simulink model "GuytonModel1972WithSubsystems_R2018_new"  (Simulink 9.1)
settings: Solver=ode23tb  StartTime=0.0  StopTime=inf  RelTol=1e-3  EnableMultiTasking=on
(part 2 of 3)

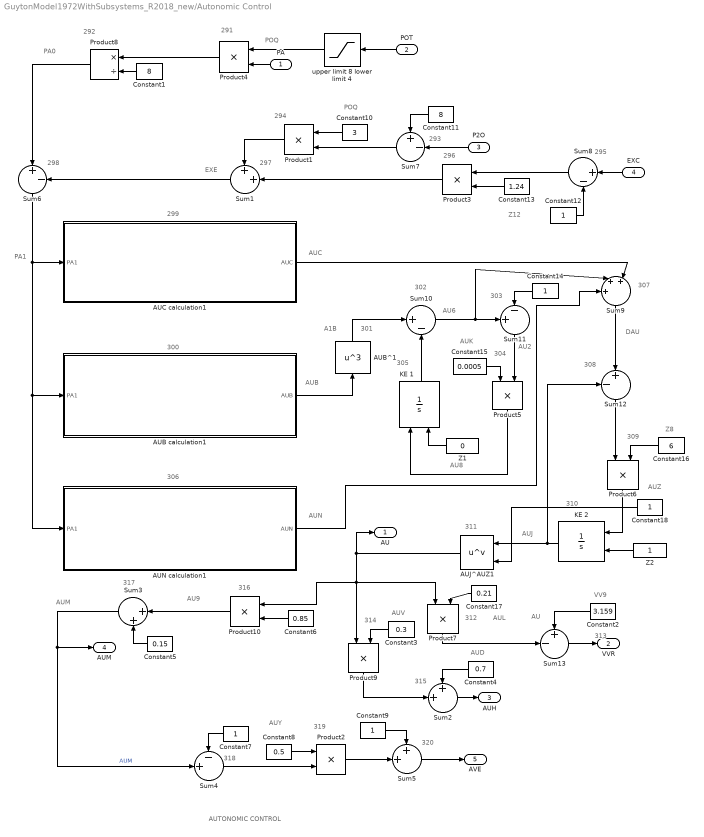
== system GuytonModel1972WithSubsystems_R2018_new/Autonomic Control ==
  note: AU
  note: AUZ
  note: PA0
  note: 306
  note: 300
  note: 294
  note: 293
  note: 305
  note: 299
  note: 297
  note: 315
  note: 295
  note: 302
  note: 309
  note: 298
  note: 314
  note: 311
  note: 301
  note: AUTONOMIC CONTROL
  note: 304
  note: 318
  note: 307
  note: 320
  note: 292
  note: AU6
  note: 316
  note: POQ
  note: DAU
  note: AU8
  note: AUK
  note: 317
  note: 291
  note: AUJ
  note: 296
  note: AUY
  note: 319
  note: 308
  note: A1B
  note: AU9
  note: 312
  note: AUV
  note: AUB
  note: 313
  note: Z12
  note: AUN
  note: AU2
  note: AUL
  note: VV9
  note: 310
  note: Z8
  note: EXE
  note: POQ
  note: 303
  note: AUC
  note: AUD
  note: PA1
  note: AUM
  PA : Inport
  POT : Inport  Port=2
  P2O : Inport  Port=3
  EXC : Inport  Port=4
  AUB calculation1 : Subsystem
      mask Display: disp('AUB CALCULATION \n\nwhen PA1<40: AUB=1.85718             \nwhen  40>PA1<170: AUB=0.014286*(170-PA1)\nwhen PA1>=170: AUB=0               \n')
  AUB^1 : Fcn  Expr=u^3
  AUC calculation1 : Subsystem
      mask Display: disp('AUC CALCULATION \n\nwhen PA1<40: AUC=1.2             \nwhen  40>PA1<80: AUC=0.03*(80-PA1)\nwhen PA1>=80: AUC=0               \n')
  AUJ^AUZ1 : Math  Operator=pow  SaturateOnIntegerOverflow=on
  AUN calculation1 : Subsystem
      mask Display: disp('AUN CALCULATION \n\nwhen PA1<50: AUN=6            \nwhen  20>PA1<50: AUN=0.2*(50-PA1)\nwhen PA1>=50: AUN=0               \n')
  Constant1 : Constant  Value=8
  Constant10 : Constant  Value=3
  Constant11 : Constant  Value=8
  Constant{7,9,12,14,18} (5 alike) : Constant
  Constant13 : Constant  Value=1.24
  Constant15 : Constant  Value=0.0005
  Constant16 : Constant  Value=6
  Constant17 : Constant  Value=0.21
  Constant2 : Constant  Value=3.159
  Constant3 : Constant  Value=0.3
  Constant4 : Constant  Value=0.7
  Constant5 : Constant  Value=0.15
  Constant6 : Constant  Value=0.85
  Constant8 : Constant  Value=0.5
  KE 1 : Integrator  InitialConditionSource=external  InitialCondition=74.7024
  KE 2 : Integrator  InitialConditionSource=external  InitialCondition=74.7024
  Product{1..7,9..10} (9 alike) : Product  SaturateOnIntegerOverflow=on  RndMeth=Zero  InputSameDT=on  OutDataTypeStr=Inherit: Same as first input
  Product8 : Product  Inputs=*/  SaturateOnIntegerOverflow=on  RndMeth=Zero  InputSameDT=on  OutDataTypeStr=Inherit: Same as first input
  Sum1 : Sum  Inputs=++|  SaturateOnIntegerOverflow=on  InputSameDT=on  OutDataTypeStr=Inherit: Same as first input
  Sum10 : Sum  Inputs=|+-  SaturateOnIntegerOverflow=on  InputSameDT=on  OutDataTypeStr=Inherit: Same as first input
  Sum11 : Sum  Inputs=+-|  SaturateOnIntegerOverflow=on  InputSameDT=on  OutDataTypeStr=Inherit: Same as first input
  Sum12 : Sum  Inputs=-+|  SaturateOnIntegerOverflow=on  InputSameDT=on  OutDataTypeStr=Inherit: Same as first input
  Sum13 : Sum  Inputs=+-|  SaturateOnIntegerOverflow=on  InputSameDT=on  OutDataTypeStr=Inherit: Same as first input
  Sum2 : Sum  Inputs=++|  SaturateOnIntegerOverflow=on  InputSameDT=on  OutDataTypeStr=Inherit: Same as first input
  Sum3 : Sum  Inputs=|++  SaturateOnIntegerOverflow=on  InputSameDT=on  OutDataTypeStr=Inherit: Same as first input
  Sum4 : Sum  Inputs=-+|  SaturateOnIntegerOverflow=on  InputSameDT=on  OutDataTypeStr=Inherit: Same as first input
  Sum5 : Sum  Inputs=++|  SaturateOnIntegerOverflow=on  InputSameDT=on  OutDataTypeStr=Inherit: Same as first input
  Sum6 : Sum  Inputs=|+-  SaturateOnIntegerOverflow=on  InputSameDT=on  OutDataTypeStr=Inherit: Same as first input
  Sum7 : Sum  Inputs=+-|  SaturateOnIntegerOverflow=on  InputSameDT=on  OutDataTypeStr=Inherit: Same as first input
  Sum8 : Sum  Inputs=|+-  SaturateOnIntegerOverflow=on  InputSameDT=on  OutDataTypeStr=Inherit: Same as first input
  Sum9 : Sum  Inputs=+++|  SaturateOnIntegerOverflow=on  InputSameDT=on  OutDataTypeStr=Inherit: Same as first input
  Z1 : Constant  Value=0
  Z2 : Constant
  "upper limit 8 lower limit 4 " : Saturate  UpperLimit=8  LowerLimit=4  LinearizeAsGain=off  ZeroCross=off
  AU : Outport
  VVR : Outport  Port=2
  AUH : Outport  Port=3
  AUM : Outport  Port=4
  AVE : Outport  Port=5
  wires:
  Sum7/1 -> Product1/2
  Sum5/1 -> AVE/1
  Sum1/1 -> Sum6/2
  Constant2/1 -> Sum13/1
  Product5/1 -> KE 1/1
  AUB^1/1 -> Sum10/1
  Constant7/1 -> Sum4/1
  Product8/1 -> Sum6/1
  Sum3/1 -> AUM/1, Sum4/2  "AUM"
  Z1/1 -> KE 1/2
  POT/1 -> "upper limit 8 lower limit 4 "/1
  Product4/1 -> Product8/1
  Constant4/1 -> Sum2/1
  Constant18/1 -> AUJ^AUZ1/2
  ? -> ?
  AUB calculation1/1(AUB) -> AUB^1/1
  Sum4/1 -> Product2/2
  Sum11/1 -> Product5/2
  Constant8/1 -> Product2/1
  Sum9/1 -> Sum12/2
  P2O/1 -> Sum7/2
  Constant1/1 -> Product8/2
  Constant9/1 -> Sum5/1
  Constant5/1 -> Sum3/2
  Product9/1 -> Sum2/2
  Constant17/1 -> Product7/2
  Product2/1 -> Sum5/2
  Z2/1 -> KE 2/2
  Constant16/1 -> Product6/2
  KE 2/1 -> Sum12/1, AUJ^AUZ1/1
  Product6/1 -> KE 2/1
  Constant3/1 -> Product9/2
  Sum12/1 -> Product6/1
  Sum6/1 -> AUC calculation1/1(PA1), AUB calculation1/1(PA1), AUN calculation1/1(PA1)
  KE 1/1 -> Sum10/2
  Product7/1 -> Sum13/2
  Constant13/1 -> Product3/2
  Constant6/1 -> Product10/2
  AUN calculation1/1(AUN) -> Sum9/1
  AUC calculation1/1(AUC) -> Sum9/3
  Constant14/1 -> Sum11/2
  Constant15/1 -> Product5/1
  Sum10/1 -> Sum11/1, Sum9/2
  Product1/1 -> Sum1/1
  Product3/1 -> Sum1/2
  AUJ^AUZ1/1 -> AU/1, Product7/1, Product9/1, Product10/1
  Sum8/1 -> Product3/1
  Product10/1 -> Sum3/1
  Constant10/1 -> Product1/1
  Constant12/1 -> Sum8/2
  "upper limit 8 lower limit 4 "/1 -> Product4/1
  Constant11/1 -> Sum7/1
  EXC/1 -> Sum8/1
  PA/1 -> Product4/2
  Sum13/1 -> VVR/1
  Sum2/1 -> AUH/1

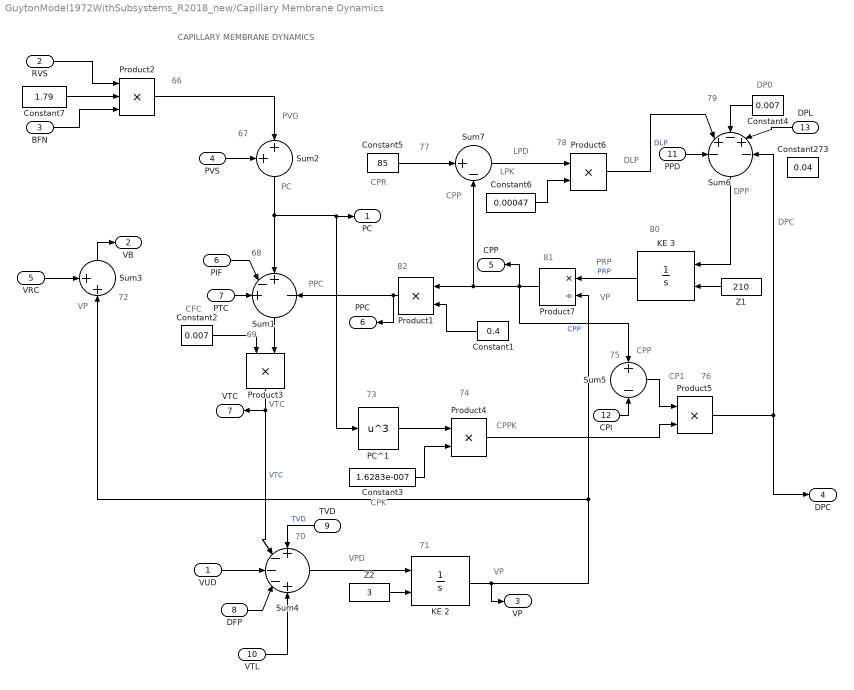
== system GuytonModel1972WithSubsystems_R2018_new/Capillary Membrane Dynamics ==
  note: VTC
  note: 72
  note: 76
  note: 73
  note: 74
  note: 71
  note: 82
  note: 66
  note: 75
  note: 70
  note: 79
  note: CAPILLARY MEMBRANE DYNAMICS
  note: 80
  note: 78
  note: 67
  note: CPPK
  note: PRP
  note: DLP
  note: 81
  note: 77
  note: VP
  note: 69
  note: VPD
  note: DP0
  note: PVG
  note: DPC
  note: CPP
  note: VP
  note: 68
  note: LPK
  note: CPR
  note: PC
  note: CP1
  note: VP
  note: PPC
  note: CPK
  note: DPP
  note: LPD
  note: CFC
  note: CPP
  VUD : Inport
  RVS : Inport  Port=2
  BFN : Inport  Port=3
  PVS : Inport  Port=4
  VRC : Inport  Port=5
  PIF : Inport  Port=6
  PTC : Inport  Port=7
  DFP : Inport  Port=8
  TVD : Inport  Port=9
  VTL : Inport  Port=10
  PPD : Inport  Port=11
  CPI : Inport  Port=12
  DPL : Inport  Port=13
  Constant1 : Constant  Value=0.4
  Constant2 : Constant  Value=0.007
  Constant273 : Constant  Value=0.04
  Constant3 : Constant  Value=1.6283e-007
  Constant4 : Constant  Value=0.007
  Constant5 : Constant  Value=85
  Constant6 : Constant  Value=0.00047
  Constant7 : Constant  Value=1.79
  KE 2 : Integrator  InitialConditionSource=external  InitialCondition=74.7024
  KE 3 : Integrator  InitialConditionSource=external  InitialCondition=74.7024
  PC^1 : Fcn  Expr=u^3
  Product{1,3..6} (5 alike) : Product  SaturateOnIntegerOverflow=on  RndMeth=Zero  InputSameDT=on  OutDataTypeStr=Inherit: Same as first input
  Product2 : Product  Inputs=3  SaturateOnIntegerOverflow=on  RndMeth=Zero  InputSameDT=on  OutDataTypeStr=Inherit: Same as first input
  Product7 : Product  Inputs=*/  SaturateOnIntegerOverflow=on  RndMeth=Zero  InputSameDT=on  OutDataTypeStr=Inherit: Same as first input
  Sum1 : Sum  Inputs=+-+|-  SaturateOnIntegerOverflow=on  InputSameDT=on  OutDataTypeStr=Inherit: Same as first input
  Sum2 : Sum  Inputs=++|  SaturateOnIntegerOverflow=on  InputSameDT=on  OutDataTypeStr=Inherit: Same as first input
  Sum3 : Sum  Inputs=++|  SaturateOnIntegerOverflow=on  InputSameDT=on  OutDataTypeStr=Inherit: Same as first input
  Sum4 : Sum  Inputs=+---+  SaturateOnIntegerOverflow=on  InputSameDT=on  OutDataTypeStr=Inherit: Same as first input
  Sum5 : Sum  Inputs=+|-  SaturateOnIntegerOverflow=on  InputSameDT=on  OutDataTypeStr=Inherit: Same as first input
  Sum6 : Sum  Inputs=-+-+-  SaturateOnIntegerOverflow=on  InputSameDT=on  OutDataTypeStr=Inherit: Same as first input
  Sum7 : Sum  Inputs=|+-  SaturateOnIntegerOverflow=on  InputSameDT=on  OutDataTypeStr=Inherit: Same as first input
  Z1 : Constant  Value=210
  Z2 : Constant  Value=3
  PC : Outport
  VB : Outport  Port=2
  VP : Outport  Port=3
  DPC : Outport  Port=4
  CPP : Outport  Port=5
  PPC : Outport  Port=6
  VTC : Outport  Port=7
  wires:
  Sum3/1 -> VB/1
  Product5/1 -> DPC/1, Sum6/5
  Product2/1 -> Sum2/2
  Product4/1 -> Product5/2
  DPL/1 -> Sum6/4
  Product7/1 -> Product1/1, Sum7/2, Sum5/1, CPP/1  "CPP"
  Sum5/1 -> Product5/1
  VRC/1 -> Sum3/1
  Z1/1 -> KE 3/2
  Constant5/1 -> Sum7/1
  Sum7/1 -> Product6/1
  Constant6/1 -> Product6/2
  Sum6/1 -> KE 3/1
  VTL/1 -> Sum4/5
  PC^1/1 -> Product4/1
  Sum4/1 -> KE 2/1
  Product6/1 -> Sum6/2  "DLP"
  Sum1/1 -> Product3/2
  Product1/1 -> PPC/1, Sum1/4
  Constant2/1 -> Product3/1
  Z2/1 -> KE 2/2
  CPI/1 -> Sum5/2
  Constant3/1 -> Product4/2
  Constant7/1 -> Product2/2
  Product3/1 -> Sum4/2, VTC/1  "VTC"
  Sum2/1 -> Sum1/3, PC/1, PC^1/1
  TVD/1 -> Sum4/1  "TVD"
  BFN/1 -> Product2/3
  KE 2/1 -> VP/1, Product7/2, Sum3/2
  PVS/1 -> Sum2/1
  KE 3/1 -> Product7/1  "PRP"
  Constant1/1 -> Product1/2
  Constant4/1 -> Sum6/3
  RVS/1 -> Product2/1
  PIF/1 -> Sum1/2
  PTC/1 -> Sum1/1
  VUD/1 -> Sum4/3
  DFP/1 -> Sum4/4
  PPD/1 -> Sum6/1

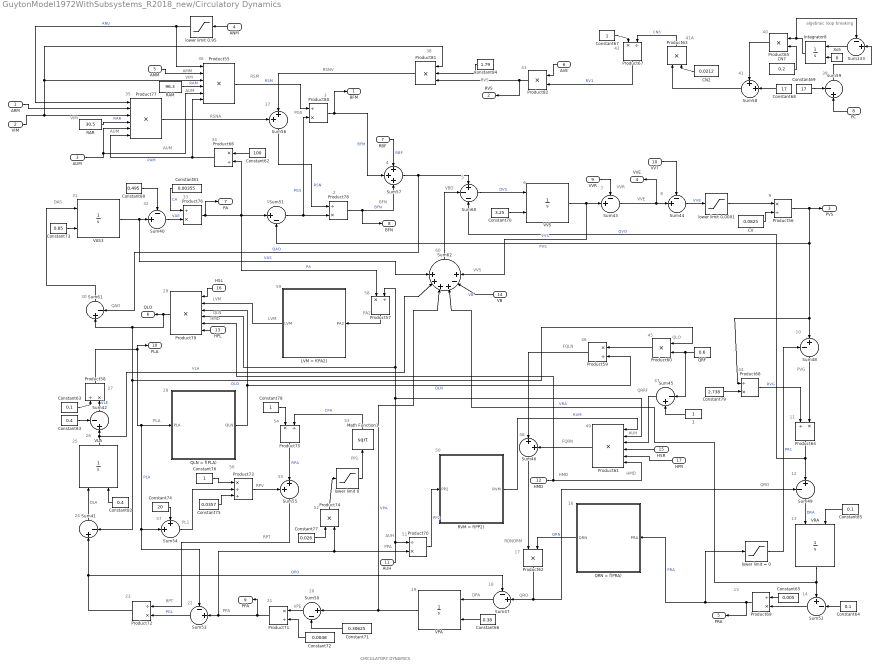
== system GuytonModel1972WithSubsystems_R2018_new/Circulatory Dynamics ==
  note: 24
  note: 25
  note: 30
  note: 58
  note: QLO
  note: AUM
  note: AUM
  note: VIM
  note: BFN
  note: 4
  note: PGS
  note: 38
  note: 39
  note: 6
  note: QLN
  note: 37
  note: AUM
  note: VBD
  note: 50
  note: VVE
  note: 16
  note: QAO
  note: 26
  note: PLA
  note: 41A
  note: 41
  note: 8
  note: 29
  note: 27
  note: 35
  note: 42
  note: 1
  note: PA2
  note: RVS
  note: 5
  note: VIM
  note: RSM
  note: 60
  note: DAS
  note: 33
  note: 31
  note: 9
  note: 59
  note: VVS
  note: 43
  note: 34
  note: 28
  note: 2
  note: 3
  note: 36
  note: 40
  note: LVM
  note: HMD
  note: RPV
  note: 46
  note: 44
  note: 7
  note: PP1
  note: 55
  note: 56
  note: 32
  note: 23
  note: 21
  note: 20
  note: 11
  note: 15
  note: 18
  note: 48
  note: QRO
  note: 22
  note: QRO
  note: VPE
  note: 54
  note: RPT
  note: 51
  note: RPT
  note: 12
  note: PL1
  note: LVM
  note: 14
  note: 45
  note: AMM
  note: 47
  note: HMD
  note: 49
  note: HMD
  note: 13
  note: VVR
  note: PPA
  note: 57
  note: AUH
  note: CIRCULATORY DYNAMICS
  note: 52
  note: 19
  note: PVG
  note: DPA
  note: RSNV
  note: AUH
  note: FQLN
  note: PPA
  note: algebraic
      | loop
      | breaking
  note: 10
  note: QRRF
  note: RDNORM
  note: 17
  note: 53
  note: FQRN
  note: RSNA
  ARM : Inport
  VIM : Inport  Port=2
  AUM : Inport  Port=3
  ANM : Inport  Port=4
  AMM : Inport  Port=5
  AVE : Inport  Port=6
  RBF : Inport  Port=7
  PC : Inport  Port=8
  VVR : Inport  Port=9
  VV7 : Inport  Port=10
  AUH : Inport  Port=11
  HMD : Inport  Port=12
  HPL : Inport  Port=13
  VB : Inport  Port=14
  HSR : Inport  Port=15
  HSL : Inport  Port=16
  HPR : Inport  Port=17
  " VAS3" : Integrator  InitialConditionSource=external
  " VLA" : Integrator  InitialConditionSource=external
  " VPA" : Integrator  InitialConditionSource=external
  " VRA" : Integrator  InitialConditionSource=external
  " VVS" : Integrator  InitialConditionSource=external
  "1 " : Constant
  CN2 : Constant  Value=0.0212
  CN7 : Constant  Value=0.2
  CV : Constant  Value=0.0825
  Constant62 : Constant  Value=100
  Constant63 : Constant  Value=0.1
  Constant64 : Constant  Value=0.1
  Constant65 : Constant  Value=0.005
  Constant66 : Constant  Value=0.38
  Constant67 : Constant
  Constant68 : Constant  Value=17
  Constant69 : Constant  Value=17
  Constant70 : Constant  Value=3.25
  Constant71 : Constant  Value=0.30625
  Constant72 : Constant  Value=0.0048
  Constant73 : Constant  Value=0.85
  Constant74 : Constant  Value=20
  Constant75 : Constant  Value=0.0357
  Constant76 : Constant
  Constant77 : Constant  Value=0.026
  Constant78 : Constant
  Constant79 : Constant  Value=2.738
  Constant80 : Constant  Value=0.495
  Constant81 : Constant  Value=0.00355
  Constant82 : Constant  Value=0.4
  Constant83 : Constant  Value=0.4
  Constant84 : Constant  Value=1.79
  Constant85 : Constant  Value=0.1
  Integrator8 : Integrator  InitialConditionSource=external
  LVM = f(PA2) : Subsystem
      mask Display:
      | plot([0 2.1 4.2 6.3 8.4 10.5 12.6 14.7 16.8 18.9 21 23.1 25.2 27.3 29.4 31.5 33.6 35.7 37.8 39.9 42 44.1 46.2 48.3 50.4 52.5 54.6 56.7 58.8 60.9 63 65.1 67.2 69.3 71.4 73.5 75.6 77.7 79.8 81.9 84 86.1 88.2 90.3 92.4 94.5 96.6 98.7 100.8 102.9 105 107.1 109.2 111.3 113.4 115.5 117.6 119.7 121.8 123.9 126 128.1 130.2 132.3 134.4 136.5 138.6 140.7 142.8 144.9 147 149.1 151.2 153.3 155.4 157.5 159.6 161.7 163.8 165.9 168 170.1 172.2 174.3 176.4 178.5 180.6 182.7 184.8 186.9 189 191.1 193.2 195.3 197.4 199.5 201.6 203.7 205.8 207.9 210 212.1 214.2 216.3 218.4 220.5 222.6 224.7 226.8 228.9 231 233.1 235.2 237.3 239.4], [1.04 1.03998 1.03993 1.03985 1.03973 1.03958 1.03941 1.0392 1.03896 1.03869 1.03839 1.03807 1.03772 1.03734 1.03693 1.03651 1.03605 1.03558 1.03508 1.03455 1.03401 1.03345 1.03286 1.03225 1.03163 1.03099 1.03033 1.02965 1.02895 1.02824 1.02752 1.02678 1.02603 1.02526 1.02443 1.0234 1.02218 1.02078 1.01923 1.01753 1.01572 1.01381 1.01181 1.00976 1.00766 1.00554 1.00341 1.00129 0.999208 0.997118 0.994998 0.992831 0.9906 0.988287 0.985875 0.983347 0.980687 0.977876 0.974898 0.971736 0.968374 0.964817 0.961055 0.95708 0.952882 0.948451 0.943777 0.93885 0.93366 0.928197 0.922452 0.916415 0.910075 0.903423 0.89645 0.889144 0.881496 0.873291 0.86413 0.854038 0.84305 0.831201 0.818528 0.805065 0.790848 0.775913 0.760295 0.744029 0.727152 0.709697 0.691702 0.673201 0.65423 0.634825 0.61502 0.594852 0.574045 0.551912 0.528467 0.503753 0.477816 0.4507 0.422449 0.393107 0.362719 0.33133 0.298983 0.265724 0.231596 0.196644 0.160913 0.124446 0.087288 0.0494838 0.0110776])
      | 
      | text(-30,0.5,'')
      | text(260,0.5,'')
      | text(25,1.15,'')
      | text(25,-0.1,'')
      | text(-25,0.05,'0')
      | text(10,-0.04,'0')
      | text(-25,1.1,'1.4')
      | text(218,-0.04,'260')
  Math Function1 : Math  Operator=sqrt  SaturateOnIntegerOverflow=on
  Product{55,61,77,79} (4 alike) : Product  Inputs=6  SaturateOnIntegerOverflow=on  RndMeth=Zero  InputSameDT=on  OutDataTypeStr=Inherit: Same as first input
  Product{56..57,59,66..67,71,75} (7 alike) : Product  Inputs=*/  SaturateOnIntegerOverflow=on  RndMeth=Zero  InputSameDT=on  OutDataTypeStr=Inherit: Same as first input
  Product{58,64,68..70,72,76,78,80} (9 alike) : Product  Inputs=/*  SaturateOnIntegerOverflow=on  RndMeth=Zero  InputSameDT=on  OutDataTypeStr=Inherit: Same as first input
  Product{60,62..63,65,74,82} (6 alike) : Product  SaturateOnIntegerOverflow=on  RndMeth=Zero  InputSameDT=on  OutDataTypeStr=Inherit: Same as first input
  Product73 : Product  Inputs=*//  SaturateOnIntegerOverflow=on  RndMeth=Zero  InputSameDT=on  OutDataTypeStr=Inherit: Same as first input
  Product81 : Product  Inputs=3  SaturateOnIntegerOverflow=on  RndMeth=Zero  InputSameDT=on  OutDataTypeStr=Inherit: Same as first input
  QLN = f(PLA) : Subsystem
      mask Display:
      | plot([     -5 -4 -3 -2 -1 0 1 2 3 4 5 6 7 8 9 10 11 12 13 14 15 16 17 18 19 20], [ 0 0.01 0.65885 2.08416 3.6 5.05 6.60577 8.16154 9.4 10.2738 10.9872 11.6 12.2245 12.8412 13.3123 13.5 13.5 13.5 13.5 13.5 13.5 13.5 13.5 13.5 13.5 13.5] )
      | 
      | 
      | text(-8,10,'')
      | text(10,-1.5,'')
      | text(22,10,'')
      | text(16,16,'')
      | text(-7,1,'0')
      | text(-5,-0.8,'-4')
      | text(-7,15,'15')
      | text(18,0,'20')
  QRF : Constant  Value=0.6
  QRN = f(PRA) : Subsystem
      mask Display:
      | plot([     -6 -5 -4 -3 -2 -1 0 1 2 3 4 5 6 7 8 9 10 11 12 13 14 15 16 17 18 19 20], [0 0.103491 0.373648 0.75 1.42618 2.6 5 7.61127 9.8 11.1961 12.1 12.6396 13.0852 13.3882 13.5 13.5 13.5 13.5 13.5 13.5 13.5 13.5 13.5 13.5 13.5 13.5 13.5])
      | 
      | 
      | 
      | text(-8,10,'')
      | text(10,-1.5,'')
      | text(22,10,'')
      | text(16,16,'')
      | text(-7,1,'0')
      | text(-5,-0.8,'-4')
      | text(-7,15,'15')
      | text(18,0,'20')
  RAM : Constant  Value=96.3
  RAR : Constant  Value=30.5
  RVM = f(PP2) : Subsystem
      mask Display:
      | plot([0 2.5 5 7.5 10 12.5 15 17.5 20 22.5 25 27.5 30 32.5 35 37.5 40 42.5 45], [1.06 1.05508 1.04813 1.03961 1.03 1.01865 1.00472 0.988437 0.97 0.947748 0.915021 0.864829 0.8 0.715601 0.608483 0.485782 0.347126 0.183428 5.55112e-017])
      | 
      | text(-8,0.5,'')
      | text(50,0.5,'')
      | text(25,1.15,'')
      | text(25,-0.1,'')
      | text(-7,0.05,'0')
      | text(-2,-0.04,'0')
      | text(-7,1.1,'1.4')
      | text(44,-0.04,'50')
  Sum{40,42..44,47..49,53,59,133} (10 alike) : Sum  Inputs=-+|  SaturateOnIntegerOverflow=on  InputSameDT=on  OutDataTypeStr=Inherit: Same as first input
  Sum{41,50..51,61} (4 alike) : Sum  Inputs=|+-  SaturateOnIntegerOverflow=on  InputSameDT=on  OutDataTypeStr=Inherit: Same as first input
  Sum45 : Sum  Inputs=|-+  SaturateOnIntegerOverflow=on  InputSameDT=on  OutDataTypeStr=Inherit: Same as first input
  Sum46 : Sum  Inputs=|++  SaturateOnIntegerOverflow=on  InputSameDT=on  OutDataTypeStr=Inherit: Same as first input
  Sum52 : Sum  Inputs=+-|  SaturateOnIntegerOverflow=on  InputSameDT=on  OutDataTypeStr=Inherit: Same as first input
  Sum{54..56,58} (4 alike) : Sum  Inputs=++|  SaturateOnIntegerOverflow=on  InputSameDT=on  OutDataTypeStr=Inherit: Same as first input
  Sum57 : Sum  Inputs=+++  SaturateOnIntegerOverflow=on  InputSameDT=on  OutDataTypeStr=Inherit: Same as first input
  Sum60 : Sum  Inputs=+--  SaturateOnIntegerOverflow=on  InputSameDT=on  OutDataTypeStr=Inherit: Same as first input
  Sum62 : Sum  Inputs=++++-+  SaturateOnIntegerOverflow=on  InputSameDT=on  OutDataTypeStr=Inherit: Same as first input
  Xo5 : Constant  Value=0  VectorParams1D=off
  "lower limit 0 " : Saturate  UpperLimit=inf  LowerLimit=0  LinearizeAsGain=off
  lower limit 0.0001 : Saturate  UpperLimit=inf  LowerLimit=0.0001  LinearizeAsGain=off
  lower limit 0.95 : Saturate  UpperLimit=inf  LowerLimit=0.95  LinearizeAsGain=off
  lower limit = 0 : Saturate  UpperLimit=inf  LowerLimit=0  LinearizeAsGain=off
  BFM : Outport
  RVS : Outport  Port=2
  PVS : Outport  Port=3
  VVE : Outport  Port=4
  PRA : Outport  Port=5
  QLO : Outport  Port=6
  PA : Outport  Port=7
  BFN : Outport  Port=8
  PPA : Outport  Port=9
  PLA : Outport  Port=10
  wires:
  "1 "/1 -> Sum45/2
  lower limit 0.95/1 -> Product77/1, Product55/1  "ANU"
  QRF/1 -> Product60/2, Sum45/1
  Product58/1 -> PLA/1, Sum54/2, Sum53/1, QLN = f(PLA)/1(PLA)  "PLA"
  Product76/1 -> PA/1, Sum51/1, Product57/1, Product66/2  "PA"
  Product59/1 -> Sum46/1
  Integrator8/1 -> Product65/1, Sum133/1
  Constant77/1 -> Product74/1
  Xo5/1 -> Integrator8/2
  Sum59/1 -> Sum133/2
  Sum46/1 -> Product62/1
  HMD/1 -> Product61/6, Product79/5
  AUH/1 -> Product57/2, Product79/4, Product61/2, Product70/1
  Sum54/1 -> Product73/2
  Sum133/1 -> Integrator8/1
  lower limit = 0/1 -> Sum48/1  "PR1"
  Product69/1 -> PRA/1, lower limit = 0/1, QRN = f(PRA)/1(PRA)  "PRA"
  Constant63/1 -> Product58/1
  Product70/1 -> RVM = f(PP2)/1(PP2)  "PP2"
  Constant71/1 -> Sum50/2
  Product71/1 -> PPA/1, Product70/2, Product74/2, Sum53/2
  " VRA"/1 -> Sum52/1, Sum62/4  "VRA"
  Constant79/1 -> Product68/2
  Constant78/1 -> Product75/1
  Sum45/1 -> Product61/3
  " VLA"/1 -> Sum42/2, Sum62/2  "VLA"
  Sum41/1 -> " VLA"/1  "DLA"
  Constant82/1 -> " VLA"/2
  "lower limit 0 "/1 -> Math Function1/1
  Sum60/1 -> " VVS"/1  "DVS"
  QLN = f(PLA)/1(QLN) -> Product59/2, Product79/3  "QLN"
  Sum58/1 -> Product63/1
  Constant68/1 -> Sum58/2
  CV/1 -> Product56/2
  Sum43/1 -> Sum44/2, VVE/1
  CN7/1 -> Product65/2
  Product65/1 -> Sum58/1
  RVM = f(PP2)/1(RVM) -> Product61/1  "RVM"
  Sum44/1 -> lower limit 0.0001/1  "VV8"
  Product80/1 -> BFM/1, Sum57/2  "BFM"
  Product67/1 -> Product82/2  "RV1"
  Product79/1 -> Sum61/1, Product60/1, Sum41/2, QLO/1  "QLO"
  ANM/1 -> lower limit 0.95/1
  Product63/1 -> Product67/2  "CN3"
  Sum40/1 -> Product76/2  "VAE"
  Product66/1 -> Product77/6, Product55/6  "PAM"
  Product81/1 -> Sum56/2
  Sum48/1 -> Product64/2
  Constant64/1 -> Sum52/2
  Constant70/1 -> " VVS"/2
  Sum52/1 -> Product69/2
  Product74/1 -> "lower limit 0 "/1
  Constant66/1 -> " VPA"/2
  Sum55/1 -> Product72/1
  Sum57/1 -> Sum60/1, Sum61/2  "QAO"
  Constant80/1 -> Sum40/1
  RAM/1 -> Product55/4  "RAM"
  Product61/1 -> Sum46/2
  Sum53/1 -> Product72/2  "PGL"
  Constant84/1 -> Product81/2
  Product68/1 -> Product64/1  "RVG"
  Product57/1 -> LVM = f(PA2)/1(PA2)
  Product78/1 -> BFN/1, Sum57/3  "BFN"
  CN2/1 -> Product63/2
  Constant67/1 -> Product67/1
  Constant81/1 -> Product76/1  "CA"
  AMM/1 -> Product55/2
  Constant65/1 -> Product69/1
  VVR/1 -> Sum43/1
  Sum51/1 -> Product78/2, Product80/2  "PGS"
  QRN = f(PRA)/1(QRN) -> Product62/2  "QRN"
  AUM/1 -> Product77/5, Product55/5
  ARM/1 -> Product77/2
  Sum62/1 -> Sum60/2
  Constant72/1 -> Product71/2
  RAR/1 -> Product77/4  "RAR"
  Constant83/1 -> Sum42/1
  Constant75/1 -> Product73/3
  Product72/1 -> Sum41/1, Sum47/1  "QPO"
  Math Function1/1 -> Product75/2  "CPA"
  Product60/1 -> Product59/1
  lower limit 0.0001/1 -> Product56/1
  Constant62/1 -> Product66/1
  Product82/1 -> RVS/1, Product81/3
  LVM = f(PA2)/1(LVM) -> Product79/2
  Sum49/1 -> " VRA"/1  "DRA"
  Constant76/1 -> Product73/1
  Sum42/1 -> Product58/2  "VLE"
  Sum50/1 -> Product71/1
  " VAS3"/1 -> Sum40/2, Sum62/1  "VAS"
  Product77/1 -> Sum56/1
  Sum47/1 -> " VPA"/1
  " VPA"/1 -> Sum50/1, Sum62/3  "VPA"
  Constant69/1 -> Sum59/1
  Product55/1 -> Product80/1  "RSM"
  Constant85/1 -> " VRA"/2
  VIM/1 -> Product77/3, Product81/1, Product55/3
  VB/1 -> Sum62/5  "VB"
  Product56/1 -> PVS/1, Sum51/2, Sum48/2, Product68/1  "PVS"
  Product64/1 -> Sum60/3, Sum49/2  "QVO"
  " VVS"/1 -> Sum62/6, Sum43/2  "VVS"
  Constant73/1 -> " VAS3"/2
  Product75/1 -> Sum55/2  "RPA"
  Sum61/1 -> " VAS3"/1
  Sum56/1 -> Product78/1  "RSN"
  Product62/1 -> Sum47/2, Sum49/1
  RBF/1 -> Sum57/1  "RBF"
  Product73/1 -> Sum55/1
  Constant74/1 -> Sum54/1
  HSL/1 -> Product79/1
  HSR/1 -> Product61/4
  HPR/1 -> Product61/5
  AVE/1 -> Product82/1
  VV7/1 -> Sum44/1
  HPL/1 -> Product79/6
  PC/1 -> Sum59/2

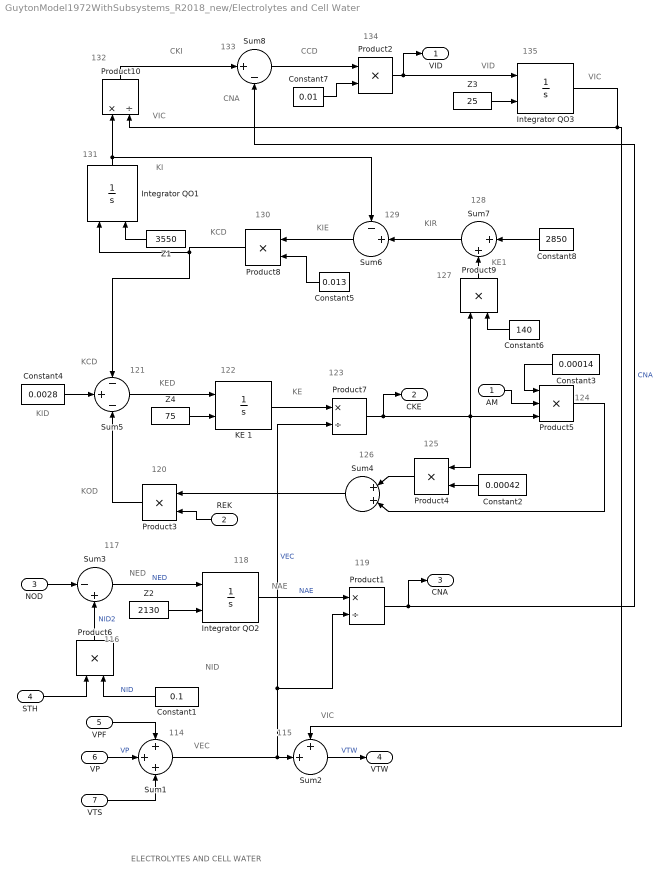
== system GuytonModel1972WithSubsystems_R2018_new/Electrolytes and Cell Water ==
  note: 132
  note: 124
  note: 129
  note: 130
  note: CKI
  note: VID
  note: KI
  note: 114
  note: VIC
  note: 122
  note: 125
  note: KE
  note: 117
  note: KCD
  note: ELECTROLYTES AND CELL WATER
  note: 115
  note: KCD
  note: 134
  note: 119
  note: KID
  note: 118
  note: VIC
  note: 121
  note: KE1
  note: 120
  note: 131
  note: CCD
  note: CNA
  note: KIE
  note: 116
  note: NAE
  note: VIC
  note: 127
  note: VEC
  note: KIR
  note: KOD
  note: NED
  note: NID
  note: 128
  note: 135
  note: 123
  note: KED
  note: 126
  note: 133
  AM : Inport
  REK : Inport  Port=2
  NOD : Inport  Port=3
  STH : Inport  Port=4
  VPF : Inport  Port=5
  VP : Inport  Port=6
  VTS : Inport  Port=7
  Constant1 : Constant  Value=0.1
  Constant2 : Constant  Value=0.00042
  Constant3 : Constant  Value=0.00014
  Constant4 : Constant  Value=0.0028
  Constant5 : Constant  Value=0.013
  Constant6 : Constant  Value=140
  Constant7 : Constant  Value=0.01
  Constant8 : Constant  Value=2850
  Integrator QO1 : Integrator  InitialConditionSource=external  InitialCondition=2403.143066
  Integrator QO2 : Integrator  InitialConditionSource=external  InitialCondition=2403.143066
  Integrator QO3 : Integrator  InitialConditionSource=external  InitialCondition=2403.143066
  KE 1 : Integrator  InitialConditionSource=external  InitialCondition=74.7024
  Product1 : Product  Inputs=*/  SaturateOnIntegerOverflow=on  RndMeth=Zero  InputSameDT=on  OutDataTypeStr=Inherit: Same as first input
  Product10 : Product  Inputs=*/  SaturateOnIntegerOverflow=on  RndMeth=Zero  InputSameDT=on  OutDataTypeStr=Inherit: Same as first input
  Product{2..4,6,8..9} (6 alike) : Product  SaturateOnIntegerOverflow=on  RndMeth=Zero  InputSameDT=on  OutDataTypeStr=Inherit: Same as first input
  Product5 : Product  Inputs=3  SaturateOnIntegerOverflow=on  RndMeth=Zero  InputSameDT=on  OutDataTypeStr=Inherit: Same as first input
  Product7 : Product  Inputs=*/  SaturateOnIntegerOverflow=on  RndMeth=Zero  InputSameDT=on  OutDataTypeStr=Inherit: Same as first input
  Sum1 : Sum  Inputs=+++  SaturateOnIntegerOverflow=on  InputSameDT=on  OutDataTypeStr=Inherit: Same as first input
  Sum2 : Sum  Inputs=++|  SaturateOnIntegerOverflow=on  InputSameDT=on  OutDataTypeStr=Inherit: Same as first input
  Sum3 : Sum  Inputs=|-+  SaturateOnIntegerOverflow=on  InputSameDT=on  OutDataTypeStr=Inherit: Same as first input
  Sum4 : Sum  Inputs=|++|  SaturateOnIntegerOverflow=on  InputSameDT=on  OutDataTypeStr=Inherit: Same as first input
  Sum5 : Sum  Inputs=-+-  SaturateOnIntegerOverflow=on  InputSameDT=on  OutDataTypeStr=Inherit: Same as first input
  Sum6 : Sum  Inputs=-+|  SaturateOnIntegerOverflow=on  InputSameDT=on  OutDataTypeStr=Inherit: Same as first input
  Sum7 : Sum  Inputs=|++  SaturateOnIntegerOverflow=on  InputSameDT=on  OutDataTypeStr=Inherit: Same as first input
  Sum8 : Sum  Inputs=|+-  SaturateOnIntegerOverflow=on  InputSameDT=on  OutDataTypeStr=Inherit: Same as first input
  Z1 : Constant  Value=3550
  Z2 : Constant  Value=2130
  Z3 : Constant  Value=25
  Z4 : Constant  Value=75
  VID : Outport
  CKE : Outport  Port=2
  CNA : Outport  Port=3
  VTW : Outport  Port=4
  wires:
  Product3/1 -> Sum5/3
  Product5/1 -> Sum4/2
  Constant4/1 -> Sum5/2
  Sum4/1 -> Product3/1
  Z3/1 -> Integrator QO3/2
  Constant6/1 -> Product9/2
  Product6/1 -> Sum3/2  "NID2"
  Z4/1 -> KE 1/2
  Constant5/1 -> Product8/2
  Constant7/1 -> Product2/2
  Product2/1 -> VID/1, Integrator QO3/1
  Constant2/1 -> Product4/2
  Constant8/1 -> Sum7/1
  Z2/1 -> Integrator QO2/2
  Sum3/1 -> Integrator QO2/1  "NED"
  Sum6/1 -> Product8/1
  Integrator QO3/1 -> Sum2/1, Product10/2
  Sum7/1 -> Sum6/2
  Integrator QO1/1 -> Sum6/1, Product10/1
  KE 1/1 -> Product7/1
  Sum5/1 -> KE 1/1
  Constant1/1 -> Product6/2  "NID"
  Z1/1 -> Integrator QO1/2
  Product7/1 -> CKE/1, Product4/1, Product5/3, Product9/1
  Constant3/1 -> Product5/1
  Product1/1 -> CNA/1, Sum8/2  "CNA"
  Sum2/1 -> VTW/1  "VTW"
  Product4/1 -> Sum4/1
  Integrator QO2/1 -> Product1/1  "NAE"
  Sum8/1 -> Product2/1
  Product10/1 -> Sum8/1
  NOD/1 -> Sum3/1
  VP/1 -> Sum1/2  "VP"
  Product8/1 -> Integrator QO1/1, Sum5/1
  Product9/1 -> Sum7/2
  Sum1/1 -> Product1/2, Product7/2, Sum2/2  "VEC"
  VTS/1 -> Sum1/3
  VPF/1 -> Sum1/1
  STH/1 -> Product6/1
  REK/1 -> Product3/2
  AM/1 -> Product5/2

== system GuytonModel1972WithSubsystems_R2018_new/Heart Hypertrophy or Deterioration ==
  note: HPR
  note: 340
  note: 347
  note: 345
  note: 342
  note: 343
  note: 348
  note: 350
  note: 351
  note: HPL
  note: DHM
  note: 352
  note: HEART HYPERTROPHY OR DETERIORATION
  note: 346
  note: 344
  note: PPA4
  note: HPL
  note: 349
  note: 341
  note: PP3
  PA : Inport
  PPA : Inport  Port=2
  HSL : Inport  Port=3
  POT : Inport  Port=4
  HSR : Inport  Port=5
  Constant1 : Constant  Value=100
  Constant2 : Constant  Value=57600
  Constant3 : Constant  Value=15
  Constant4 : Constant  Value=57600
  Constant5 : Constant  Value=6
  Constant6 : Constant  Value=0.0025
  KE 1 : Integrator  InitialConditionSource=external  InitialCondition=74.7024
  KE 2 : Integrator  InitialConditionSource=external  InitialCondition=74.7024
  KE 3 : Integrator  InitialConditionSource=external  InitialCondition=74.7024
  PA4^0.1 : Fcn  Expr=u^0.625
  PP3^0.2 : Fcn  Expr=u^0.625
  Product1 : Product  Inputs=*/  SaturateOnIntegerOverflow=on  RndMeth=Zero  InputSameDT=on  OutDataTypeStr=Inherit: Same as first input
  Product2 : Product  Inputs=/*/  SaturateOnIntegerOverflow=on  RndMeth=Zero  InputSameDT=on  OutDataTypeStr=Inherit: Same as first input
  Product3 : Product  Inputs=*/  SaturateOnIntegerOverflow=on  RndMeth=Zero  InputSameDT=on  OutDataTypeStr=Inherit: Same as first input
  Product4 : Product  SaturateOnIntegerOverflow=on  RndMeth=Zero  InputSameDT=on  OutDataTypeStr=Inherit: Same as first input
  Product5 : Product  Inputs=/*/  SaturateOnIntegerOverflow=on  RndMeth=Zero  InputSameDT=on  OutDataTypeStr=Inherit: Same as first input
  Sum1 : Sum  Inputs=|+-  SaturateOnIntegerOverflow=on  InputSameDT=on  OutDataTypeStr=Inherit: Same as first input
  Sum2 : Sum  Inputs=|+-  SaturateOnIntegerOverflow=on  InputSameDT=on  OutDataTypeStr=Inherit: Same as first input
  Sum3 : Sum  Inputs=|+-  SaturateOnIntegerOverflow=on  InputSameDT=on  OutDataTypeStr=Inherit: Same as first input
  Z1 : Constant
  Z2 : Constant
  Z3 : Constant
  upper limit 1 : Saturate  UpperLimit=1  LowerLimit=0  LinearizeAsGain=off
  HPR : Outport
  HPL : Outport  Port=2
  HMD : Outport  Port=3
  wires:
  HSR/1 -> Product2/1
  HSL/1 -> Product5/1
  PP3^0.2/1 -> Sum1/1
  Product2/1 -> PP3^0.2/1
  POT/1 -> Sum2/1
  Constant4/1 -> Product3/2
  Sum3/1 -> Product1/1
  KE 3/1 -> Sum1/2, HPR/1
  Constant2/1 -> Product1/2
  KE 2/1 -> HPL/1, Sum3/2
  Product4/1 -> KE 1/1
  Constant3/1 -> Product2/3
  Sum2/1 -> Product4/1
  Product3/1 -> KE 3/1
  Constant5/1 -> Sum2/2
  Z2/1 -> KE 1/2
  Sum1/1 -> Product3/1
  Z1/1 -> KE 3/2
  KE 1/1 -> upper limit 1/1
  Constant1/1 -> Product5/3
  Constant6/1 -> Product4/2
  Product1/1 -> KE 2/1
  Z3/1 -> KE 2/2
  PA4^0.1/1 -> Sum3/1
  Product5/1 -> PA4^0.1/1
  PA/1 -> Product5/2
  PPA/1 -> Product2/2
  upper limit 1/1 -> HMD/1

== system GuytonModel1972WithSubsystems_R2018_new/Heart Rate and Stroke Volume ==
  note: HR
  note: HRPRA
  note: HRN
  note: HRHMD
  note: AU
  note: 327
  note: HMD
  note: 325
  note: HEART RATE AND STROKE VOLUME
  note: 328
  note: HR
  note: 322
  note: HRAU
  note: 326
  note: PRA
  note: 323
  note: QLO
  note: 321
  note: HR
  note: SVO
  note: 324
  AU : Inport
  HMD : Inport  Port=2
  PRA : Inport  Port=3
  QLO : Inport  Port=4
  Constant1 : Constant  Value=2
  Constant2 : Constant  Value=40
  Constant3 : Constant
  Constant4 : Constant  Value=0.5
  Constant5 : Constant  Value=32
  Constant6 : Constant
  Product{1..4} (4 alike) : Product  SaturateOnIntegerOverflow=on  RndMeth=Zero  InputSameDT=on  OutDataTypeStr=Inherit: Same as first input
  Product5 : Product  Inputs=*/  SaturateOnIntegerOverflow=on  RndMeth=Zero  InputSameDT=on  OutDataTypeStr=Inherit: Same as first input
  Sum1 : Sum  Inputs=|++  SaturateOnIntegerOverflow=on  InputSameDT=on  OutDataTypeStr=Inherit: Same as first input
  Sum2 : Sum  Inputs=+++  SaturateOnIntegerOverflow=on  InputSameDT=on  OutDataTypeStr=Inherit: Same as first input
  Sum3 : Sum  Inputs=|+-  SaturateOnIntegerOverflow=on  InputSameDT=on  OutDataTypeStr=Inherit: Same as first input
  SVO : Outport
  HR : Outport  Port=2
  wires:
  Constant3/1 -> Sum3/2
  HMD/1 -> Sum3/1
  AU/1 -> Product2/2
  Product5/1 -> SVO/1  "SVO"
  Sum1/1 -> Product1/2
  QLO/1 -> Product5/1
  Product2/1 -> Sum2/3
  Constant2/1 -> Product2/1
  Product3/1 -> Sum1/2
  Product4/1 -> Sum2/2
  Product1/1 -> HR/1, Product5/2
  PRA/1 -> Product4/2
  Sum2/1 -> Product1/1
  Constant1/1 -> Product4/1
  Sum3/1 -> Product3/1
  Constant4/1 -> Product3/2
  Constant5/1 -> Sum2/1
  Constant6/1 -> Sum1/1

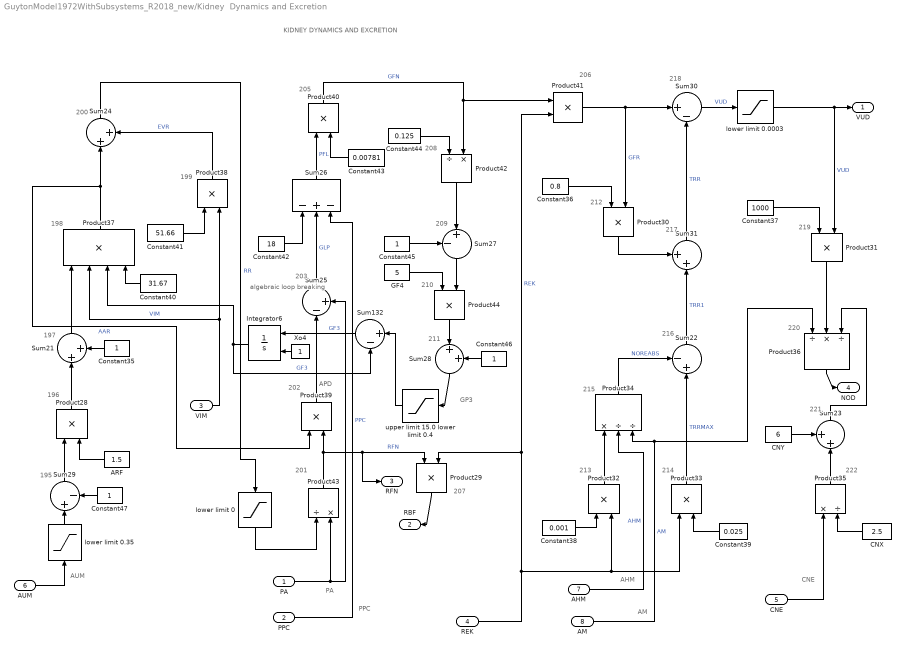
== system GuytonModel1972WithSubsystems_R2018_new/Kidney  Dynamics and Excretion ==
  note: PPC
  note: AUM
  note: CNE
  note: GP3
  note: algebraic
      | loop
      | breaking
  note: 209
  note: KIDNEY DYNAMICS AND EXCRETION
  note: AHM
  note: 218
  note: 198
  note: 201
  note: 221
  note: AM
  note: 213
  note: 220
  note: 196
  note: 219
  note: 206
  note: 211
  note: APD
  note: 199
  note: 208
  note: 217
  note: 212
  note: 195
  note: 210
  note: 200
  note: 197
  note: 216
  note: 203
  note: 222
  note: 214
  note: PA
  note: 202
  note: 205
  note: 207
  note: 215
  PA : Inport
  PPC : Inport  Port=2
  VIM : Inport  Port=3
  REK : Inport  Port=4
  CNE : Inport  Port=5
  AUM : Inport  Port=6
  AHM : Inport  Port=7
  AM : Inport  Port=8
  " lower limit 0" : Saturate  UpperLimit=inf  LowerLimit=0.0001  LinearizeAsGain=off
  " lower limit 0.35" : Saturate  UpperLimit=inf  LowerLimit=0.35  LinearizeAsGain=off
  ARF : Constant  Value=1.5
  CNX : Constant  Value=2.5
  CNY : Constant  Value=6
  Constant{35,45..47} (4 alike) : Constant
  Constant36 : Constant  Value=0.8
  Constant37 : Constant  Value=1000
  Constant38 : Constant  Value=0.001
  Constant39 : Constant  Value=0.025
  Constant40 : Constant  Value=31.67
  Constant41 : Constant  Value=51.66
  Constant42 : Constant  Value=18
  Constant43 : Constant  Value=0.00781
  Constant44 : Constant  Value=0.125
  GF4 : Constant  Value=5
  Integrator6 : Integrator  InitialConditionSource=external  InitialCondition=1
  Product{28..33,38..41,44} (11 alike) : Product  SaturateOnIntegerOverflow=on  RndMeth=Zero  InputSameDT=on  OutDataTypeStr=Inherit: Same as first input
  Product34 : Product  Inputs=*//  SaturateOnIntegerOverflow=on  RndMeth=Zero  InputSameDT=on  OutDataTypeStr=Inherit: Same as first input
  Product35 : Product  Inputs=*/  SaturateOnIntegerOverflow=on  RndMeth=Zero  InputSameDT=on  OutDataTypeStr=Inherit: Same as first input
  Product36 : Product  Inputs=/*/  SaturateOnIntegerOverflow=on  RndMeth=Zero  InputSameDT=on  OutDataTypeStr=Inherit: Same as first input
  Product37 : Product  Inputs=4  SaturateOnIntegerOverflow=on  RndMeth=Zero  InputSameDT=on  OutDataTypeStr=Inherit: Same as first input
  Product42 : Product  Inputs=/*  SaturateOnIntegerOverflow=on  RndMeth=Zero  InputSameDT=on  OutDataTypeStr=Inherit: Same as first input
  Product43 : Product  Inputs=/*  SaturateOnIntegerOverflow=on  RndMeth=Zero  InputSameDT=on  OutDataTypeStr=Inherit: Same as first input
  Sum132 : Sum  Inputs=|+-  SaturateOnIntegerOverflow=on  InputSameDT=on  OutDataTypeStr=Inherit: Same as first input
  Sum21 : Sum  Inputs=|++  SaturateOnIntegerOverflow=on  InputSameDT=on  OutDataTypeStr=Inherit: Same as first input
  Sum22 : Sum  Inputs=-+|  SaturateOnIntegerOverflow=on  InputSameDT=on  OutDataTypeStr=Inherit: Same as first input
  Sum23 : Sum  Inputs=++|  SaturateOnIntegerOverflow=on  InputSameDT=on  OutDataTypeStr=Inherit: Same as first input
  Sum24 : Sum  Inputs=|++  SaturateOnIntegerOverflow=on  InputSameDT=on  OutDataTypeStr=Inherit: Same as first input
  Sum25 : Sum  Inputs=|-+  SaturateOnIntegerOverflow=on  InputSameDT=on  OutDataTypeStr=Inherit: Same as first input
  Sum26 : Sum  Inputs=-+-  SaturateOnIntegerOverflow=on  InputSameDT=on  OutDataTypeStr=Inherit: Same as first input
  Sum27 : Sum  Inputs=-+|  SaturateOnIntegerOverflow=on  InputSameDT=on  OutDataTypeStr=Inherit: Same as first input
  Sum28 : Sum  Inputs=|++  SaturateOnIntegerOverflow=on  InputSameDT=on  OutDataTypeStr=Inherit: Same as first input
  Sum29 : Sum  Inputs=|+-  SaturateOnIntegerOverflow=on  InputSameDT=on  OutDataTypeStr=Inherit: Same as first input
  Sum30 : Sum  Inputs=|+-  SaturateOnIntegerOverflow=on  InputSameDT=on  OutDataTypeStr=Inherit: Same as first input
  Sum31 : Sum  Inputs=++|  SaturateOnIntegerOverflow=on  InputSameDT=on  OutDataTypeStr=Inherit: Same as first input
  Xo4 : Constant  VectorParams1D=off
  lower limit 0.0003 : Saturate  UpperLimit=inf  LowerLimit=0.0003  LinearizeAsGain=off
  upper limit 15.0 lower limit 0.4 : Saturate  UpperLimit=15  LowerLimit=0.4  LinearizeAsGain=off
  VUD : Outport
  RBF : Outport  Port=2
  RFN : Outport  Port=3
  NOD : Outport  Port=4
  wires:
  " lower limit 0"/1 -> Product43/1
  Product44/1 -> Sum28/1
  upper limit 15.0 lower limit 0.4/1 -> Sum132/1
  Sum132/1 -> Integrator6/1  "GF3"
  Integrator6/1 -> Sum132/2, Product37/3  "GF3"
  REK/1 -> Product41/2, Product29/2, Product32/2, Product33/1  "REK"
  Constant36/1 -> Product30/1
  Product32/1 -> Product34/1
  PA/1 -> Sum25/2, Product43/2
  Product38/1 -> Sum24/2  "EVR"
  Constant45/1 -> Sum27/1
  Product43/1 -> Product39/2, RFN/1, Product29/1  "RFN"
  Constant46/1 -> Sum28/2
  Product28/1 -> Sum21/1
  AHM/1 -> Product34/2  "AHM"
  Product39/1 -> Sum25/1
  Sum23/1 -> Product36/3
  Constant38/1 -> Product32/1
  Product41/1 -> Product30/2, Sum30/1  "GFR"
  Product37/1 -> Product39/1, Sum24/1  "AAR"
  Sum28/1 -> upper limit 15.0 lower limit 0.4/1
  Constant44/1 -> Product42/1
  Product33/1 -> Sum22/2  "TRRMAX"
  Product30/1 -> Sum31/1
  Product42/1 -> Sum27/2
  Sum31/1 -> Sum30/2  "TRR"
  Product31/1 -> Product36/2
  Constant43/1 -> Product40/2
  CNY/1 -> Sum23/1
  Constant47/1 -> Sum29/2
  Sum30/1 -> lower limit 0.0003/1  "VUD"
  Sum22/1 -> Sum31/2  "TRR1"
  lower limit 0.0003/1 -> VUD/1, Product31/2  "VUD"
  Product40/1 -> Product41/1, Product42/2  "GFN"
  Constant37/1 -> Product31/1
  CNX/1 -> Product35/2
  " lower limit 0.35"/1 -> Sum29/1
  Constant42/1 -> Sum26/1
  Sum25/1 -> Sum26/2  "GLP"
  Sum26/1 -> Product40/1  "PFL"
  Product34/1 -> Sum22/1  "NOREABS"
  VIM/1 -> Product38/2, Product37/2  "VIM"
  Xo4/1 -> Integrator6/2
  AM/1 -> Product34/3, Product36/1  "AM"
  PPC/1 -> Sum26/3  "PPC"
  Product35/1 -> Sum23/2
  Sum21/1 -> Product37/1
  Sum29/1 -> Product28/1
  Sum24/1 -> " lower limit 0"/1  "RR"
  CNE/1 -> Product35/1
  Constant40/1 -> Product37/4
  Constant41/1 -> Product38/1
  Sum27/1 -> Product44/2
  Constant35/1 -> Sum21/2
  Constant39/1 -> Product33/2
  ARF/1 -> Product28/2
  GF4/1 -> Product44/1
  AUM/1 -> " lower limit 0.35"/1
  Product36/1 -> NOD/1
  Product29/1 -> RBF/1

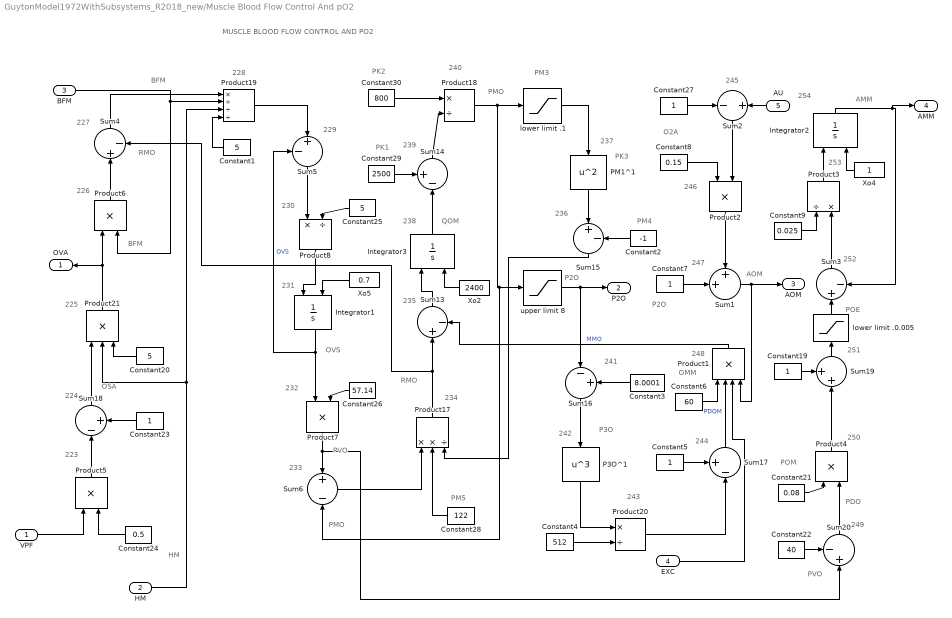
== system GuytonModel1972WithSubsystems_R2018_new/Muscle Blood Flow Control And pO2 ==
  note: PM5
  note: POM
  note: 244
  note: AMM
  note: 249
  note: PM3
  note: POE
  note: PK1
  note: RMO
  note: 251
  note: 236
  note: 254
  note: 240
  note: 245
  note: P2O
  note: 250
  note: P2O
  note: 252
  note: PMO
  note: OSA
  note: 253
  note: PM4
  note: PDO
  note: 247
  note: 237
  note: 239
  note: PK3
  note: PMO
  note: 246
  note: RMO
  note: BFM
  note: 243
  note: 242
  note: BFM
  note: PVO
  note: HM
  note: AOM
  note: OMM
  note: MUSCLE BLOOD FLOW CONTROL AND PO2
  note: 223
  note: 229
  note: 235
  note: 232
  note: O2A
  note: 227
  note: QOM
  note: 241
  note: PVO
  note: 228
  note: 248
  note: 226
  note: 225
  note: 231
  note: OVS
  note: 230
  note: 238
  note: P3O
  note: 234
  note: 224
  note: 233
  note: PK2
  VPF : Inport
  HM : Inport  Port=2
  BFM : Inport  Port=3
  EXC : Inport  Port=4
  AU : Inport  Port=5
  Constant1 : Constant  Value=5
  Constant{5,7,19,23,27} (5 alike) : Constant
  Constant2 : Constant  Value=-1
  Constant20 : Constant  Value=5
  Constant21 : Constant  Value=0.08
  Constant22 : Constant  Value=40
  Constant24 : Constant  Value=0.5
  Constant25 : Constant  Value=5
  Constant26 : Constant  Value=57.14
  Constant28 : Constant  Value=122
  Constant29 : Constant  Value=2500
  Constant3 : Constant  Value=8.0001
  Constant30 : Constant  Value=800
  Constant4 : Constant  Value=512
  Constant6 : Constant  Value=60
  Constant8 : Constant  Value=0.15
  Constant9 : Constant  Value=0.025
  Integrator1 : Integrator  InitialConditionSource=external
  Integrator2 : Integrator  InitialConditionSource=external  InitialCondition=2399.9633789
  Integrator3 : Integrator  InitialConditionSource=external  InitialCondition=2399.9633789
  P3O^1 : Fcn  Expr=u^3
  PM1^1 : Fcn  Expr=u^2
  Product1 : Product  Inputs=4  SaturateOnIntegerOverflow=on  RndMeth=Zero  InputSameDT=on  OutDataTypeStr=Inherit: Same as first input
  Product17 : Product  Inputs=**/  SaturateOnIntegerOverflow=on  RndMeth=Zero  InputSameDT=on  OutDataTypeStr=Inherit: Same as first input
  Product18 : Product  Inputs=*/  SaturateOnIntegerOverflow=on  RndMeth=Zero  InputSameDT=on  OutDataTypeStr=Inherit: Same as first input
  Product19 : Product  Inputs=*///  SaturateOnIntegerOverflow=on  RndMeth=Zero  InputSameDT=on  OutDataTypeStr=Inherit: Same as first input
  Product{2,4..7} (5 alike) : Product  SaturateOnIntegerOverflow=on  RndMeth=Zero  InputSameDT=on  OutDataTypeStr=Inherit: Same as first input
  Product20 : Product  Inputs=*/  SaturateOnIntegerOverflow=on  RndMeth=Zero  InputSameDT=on  OutDataTypeStr=Inherit: Same as first input
  Product21 : Product  Inputs=3  SaturateOnIntegerOverflow=on  RndMeth=Zero  InputSameDT=on  OutDataTypeStr=Inherit: Same as first input
  Product3 : Product  Inputs=/*  SaturateOnIntegerOverflow=on  RndMeth=Zero  InputSameDT=on  OutDataTypeStr=Inherit: Same as first input
  Product8 : Product  Inputs=*/  SaturateOnIntegerOverflow=on  RndMeth=Zero  InputSameDT=on  OutDataTypeStr=Inherit: Same as first input
  Sum1 : Sum  Inputs=++|  SaturateOnIntegerOverflow=on  InputSameDT=on  OutDataTypeStr=Inherit: Same as first input
  Sum{3..4,13,15} (4 alike) : Sum  Inputs=|+-  SaturateOnIntegerOverflow=on  InputSameDT=on  OutDataTypeStr=Inherit: Same as first input
  Sum14 : Sum  Inputs=+-|  SaturateOnIntegerOverflow=on  InputSameDT=on  OutDataTypeStr=Inherit: Same as first input
  Sum16 : Sum  Inputs=|-+  SaturateOnIntegerOverflow=on  InputSameDT=on  OutDataTypeStr=Inherit: Same as first input
  Sum17 : Sum  Inputs=+-|  SaturateOnIntegerOverflow=on  InputSameDT=on  OutDataTypeStr=Inherit: Same as first input
  Sum18 : Sum  Inputs=|-+  SaturateOnIntegerOverflow=on  InputSameDT=on  OutDataTypeStr=Inherit: Same as first input
  Sum19 : Sum  Inputs=++|  SaturateOnIntegerOverflow=on  InputSameDT=on  OutDataTypeStr=Inherit: Same as first input
  Sum2 : Sum  Inputs=-|+  SaturateOnIntegerOverflow=on  InputSameDT=on  OutDataTypeStr=Inherit: Same as first input
  Sum20 : Sum  Inputs=-+|  SaturateOnIntegerOverflow=on  InputSameDT=on  OutDataTypeStr=Inherit: Same as first input
  Sum5 : Sum  Inputs=-+|  SaturateOnIntegerOverflow=on  InputSameDT=on  OutDataTypeStr=Inherit: Same as first input
  Sum6 : Sum  Inputs=+|-  SaturateOnIntegerOverflow=on  InputSameDT=on  OutDataTypeStr=Inherit: Same as first input
  Xo2 : Constant  Value=2400  VectorParams1D=off
  Xo4 : Constant  VectorParams1D=off
  Xo5 : Constant  Value=0.7  VectorParams1D=off
  lower limit .0.005 : Saturate  UpperLimit=inf  LowerLimit=0.005  LinearizeAsGain=off
  lower limit .1 : Saturate  UpperLimit=inf  LowerLimit=0.001  LinearizeAsGain=off
  "upper limit 8 " : Saturate  UpperLimit=8  LowerLimit=0  LinearizeAsGain=off
  OVA : Outport
  P2O : Outport  Port=2
  AOM : Outport  Port=3
  AMM : Outport  Port=4
  wires:
  Constant1/1 -> Product19/4
  PM1^1/1 -> Sum15/1
  Product2/1 -> Sum1/1
  Integrator2/1 -> AMM/1, Sum3/2
  Sum13/1 -> Integrator3/1
  Constant4/1 -> Product20/2
  Constant28/1 -> Product17/2
  Constant25/1 -> Product8/2
  Sum17/1 -> Product1/2  "PDOM"
  Product1/1 -> Sum13/2  "MMO"
  Product5/1 -> Sum18/1
  Constant27/1 -> Sum2/1
  Constant2/1 -> Sum15/2
  Sum16/1 -> P3O^1/1
  Constant29/1 -> Sum14/1
  Product21/1 -> OVA/1, Product6/1
  Sum20/1 -> Product4/2
  Constant24/1 -> Product5/2
  Xo4/1 -> Integrator2/2
  Constant21/1 -> Product4/1
  Constant30/1 -> Product18/1
  Xo2/1 -> Integrator3/2
  Sum15/1 -> Product17/3
  lower limit .0.005/1 -> Sum3/1
  Constant8/1 -> Product2/1
  Product4/1 -> Sum19/2
  Constant19/1 -> Sum19/1
  P3O^1/1 -> Product20/1
  Product18/1 -> lower limit .1/1, Sum6/2, "upper limit 8 "/1
  Sum2/1 -> Product2/2
  Product17/1 -> Sum4/2, Sum13/1
  Constant3/1 -> Sum16/2
  Product20/1 -> Sum17/2
  Constant9/1 -> Product3/1
  Constant6/1 -> Product1/1
  Constant5/1 -> Sum17/1
  Sum3/1 -> Product3/2
  Integrator3/1 -> Sum14/2
  Product3/1 -> Integrator2/1
  Sum5/1 -> Product8/1
  Product19/1 -> Sum5/2
  Sum1/1 -> AOM/1, Product1/4
  Constant26/1 -> Product7/2
  Sum6/1 -> Product17/1
  Product7/1 -> Sum6/1, Sum20/2
  Sum18/1 -> Product21/1
  Xo5/1 -> Integrator1/2
  Product8/1 -> Integrator1/1
  Sum14/1 -> Product18/2
  Integrator1/1 -> Sum5/1, Product7/1  "OVS"
  Constant7/1 -> Sum1/2
  Constant23/1 -> Sum18/2
  Product6/1 -> Sum4/1
  lower limit .1/1 -> PM1^1/1
  Constant22/1 -> Sum20/1
  "upper limit 8 "/1 -> P2O/1, Sum16/1
  Sum19/1 -> lower limit .0.005/1
  Sum4/1 -> Product19/1
  Constant20/1 -> Product21/3
  VPF/1 -> Product5/1
  EXC/1 -> Product1/3
  AU/1 -> Sum2/2
  BFM/1 -> Product6/2, Product19/2
  HM/1 -> Product19/3, Product21/2

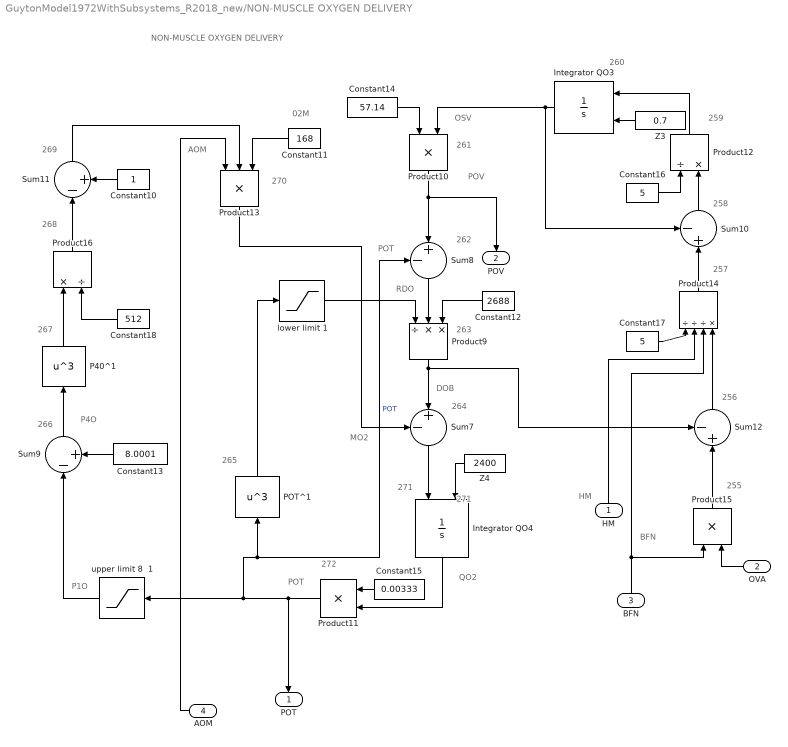
== system GuytonModel1972WithSubsystems_R2018_new/NON-MUSCLE OXYGEN DELIVERY ==
  note: 269
  note: 260
  note: 268
  note: 264
  note: BFN
  note: 267
  note: 259
  note: 270
  note: HM
  note: 271
  note: 257
  note: 258
  note: 261
  note: NON-MUSCLE OXYGEN DELIVERY
  note: 262
  note: 266
  note: 263
  note: 272
  note: 256
  note: 255
  note: POV
  note: OSV
  note: POT
  note: RDO
  note: DOB
  note: P1O
  note: 02M
  note: P4O
  note: MO2
  note: 265
  note: QO2
  note: 271
  note: AOM
  note: POT
  HM : Inport
  OVA : Inport  Port=2
  BFN : Inport  Port=3
  AOM : Inport  Port=4
  Constant10 : Constant
  Constant11 : Constant  Value=168
  Constant12 : Constant  Value=2688
  Constant13 : Constant  Value=8.0001
  Constant14 : Constant  Value=57.14
  Constant15 : Constant  Value=0.00333
  Constant16 : Constant  Value=5
  Constant17 : Constant  Value=5
  Constant18 : Constant  Value=512
  Integrator QO3 : Integrator  InitialConditionSource=external  InitialCondition=2403.143066
  Integrator QO4 : Integrator  InitialConditionSource=external  InitialCondition=2403.143066
  P40^1 : Fcn  Expr=u^3
  POT^1 : Fcn  Expr=u^3
  Product10 : Product  SaturateOnIntegerOverflow=on  RndMeth=Zero  InputSameDT=on  OutDataTypeStr=Inherit: Same as first input
  Product11 : Product  SaturateOnIntegerOverflow=on  RndMeth=Zero  InputSameDT=on  OutDataTypeStr=Inherit: Same as first input
  Product12 : Product  Inputs=/*  SaturateOnIntegerOverflow=on  RndMeth=Zero  InputSameDT=on  OutDataTypeStr=Inherit: Same as first input
  Product13 : Product  Inputs=3  SaturateOnIntegerOverflow=on  RndMeth=Zero  InputSameDT=on  OutDataTypeStr=Inherit: Same as first input
  Product14 : Product  Inputs=///*  SaturateOnIntegerOverflow=on  RndMeth=Zero  InputSameDT=on  OutDataTypeStr=Inherit: Same as first input
  Product15 : Product  SaturateOnIntegerOverflow=on  RndMeth=Zero  InputSameDT=on  OutDataTypeStr=Inherit: Same as first input
  Product16 : Product  Inputs=*/  SaturateOnIntegerOverflow=on  RndMeth=Zero  InputSameDT=on  OutDataTypeStr=Inherit: Same as first input
  Product9 : Product  Inputs=/**  SaturateOnIntegerOverflow=on  RndMeth=Zero  InputSameDT=on  OutDataTypeStr=Inherit: Same as first input
  Sum{7..8,10,12} (4 alike) : Sum  Inputs=-+|  SaturateOnIntegerOverflow=on  InputSameDT=on  OutDataTypeStr=Inherit: Same as first input
  Sum11 : Sum  Inputs=|-+  SaturateOnIntegerOverflow=on  InputSameDT=on  OutDataTypeStr=Inherit: Same as first input
  Sum9 : Sum  Inputs=|-+  SaturateOnIntegerOverflow=on  InputSameDT=on  OutDataTypeStr=Inherit: Same as first input
  Z3 : Constant  Value=0.7
  Z4 : Constant  Value=2400
  lower limit 1 : Saturate  UpperLimit=inf  LowerLimit=50  LinearizeAsGain=off
  upper limit 8  1 : Saturate  UpperLimit=8  LowerLimit=-inf  LinearizeAsGain=off  ZeroCross=off
  POT : Outport
  POV : Outport  Port=2
  wires:
  Integrator QO3/1 -> Sum10/1, Product10/2
  Sum12/1 -> Product14/4
  Product11/1 -> POT/1, POT^1/1, Sum8/1, upper limit 8  1/1  "POT"
  HM/1 -> Product14/2
  Product12/1 -> Integrator QO3/1
  Product10/1 -> POV/1, Sum8/2
  OVA/1 -> Product15/2
  Constant11/1 -> Product13/3
  Product9/1 -> Sum7/2, Sum12/1
  Product15/1 -> Sum12/2
  Sum7/1 -> Integrator QO4/1
  AOM/1 -> Product13/1
  Sum11/1 -> Product13/2
  Sum9/1 -> P40^1/1
  Z3/1 -> Integrator QO3/2
  upper limit 8  1/1 -> Sum9/1
  Constant14/1 -> Product10/1
  Sum8/1 -> Product9/2
  Product13/1 -> Sum7/1
  P40^1/1 -> Product16/1
  Constant13/1 -> Sum9/2
  lower limit 1/1 -> Product9/1
  Sum10/1 -> Product12/2
  Integrator QO4/1 -> Product11/2
  Constant10/1 -> Sum11/2
  Constant17/1 -> Product14/1
  Product16/1 -> Sum11/1
  Constant18/1 -> Product16/2
  Constant16/1 -> Product12/1
  BFN/1 -> Product15/1, Product14/3
  Product14/1 -> Sum10/2
  Z4/1 -> Integrator QO4/2
  Constant15/1 -> Product11/1
  Constant12/1 -> Product9/3
  POT^1/1 -> lower limit 1/1
